simulink model "controller"  (R2023b)
settings: Solver=FixedStepAuto  StartTime=0.0  StopTime=10.0  FixedStep=1/100  RelTol=1e-3
values from neighbouring files (symbols this model uses):
  MAX_TORQUE = 80    [init_fn.m]
  MAX_TORQUE_REVERSE = 40    [init_fn.m]
undefined symbols (not defined in the file or in its folder): MAX_SPEED_BACKWARD, MAX_SPEED_FORWARD
settings Model: Creator=DAUIN-Win10  LastModifiedBy=anton
settings OptimizationCC: ReuseModelBlockBuffer=off
settings DebuggingCC: UnconnectedInputMsg=warning  UnconnectedOutputMsg=warning  UnconnectedLineMsg=warning  UnderSpecifiedDimensionMsg=error
settings ModelReferenceCC: EnableRefExpFcnMdlSchedulingChecks=on
settings RTWCC: DLArmComputeVersion=19.05

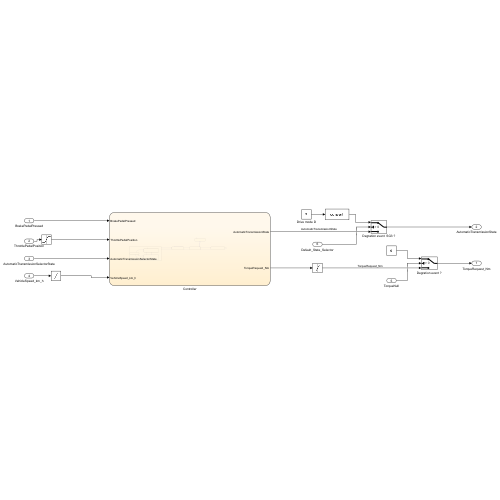
[thumbnail: Simulink's stored preview of the top-level diagram]
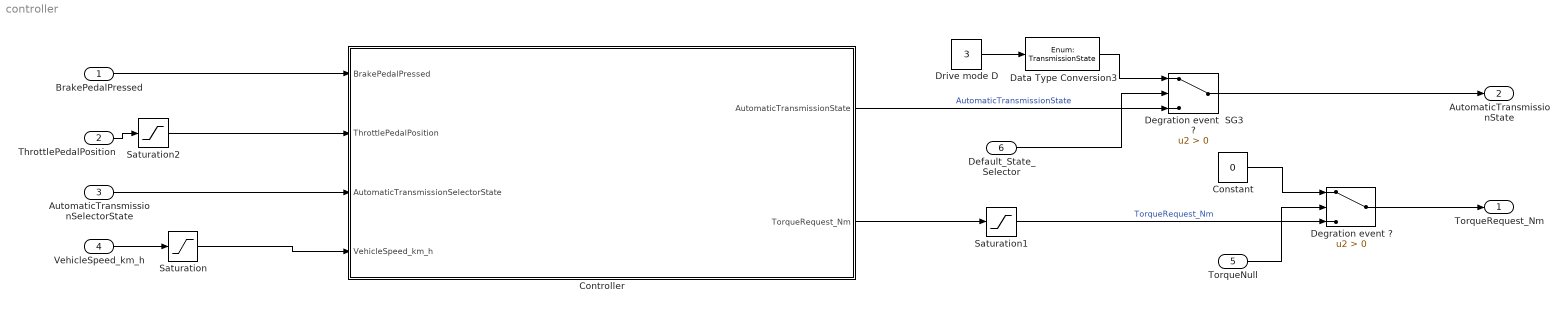
== system controller ==
  BrakePedalPressed : Inport  OutDataTypeStr=boolean
  ThrottlePedalPosition : Inport  Port=2  OutDataTypeStr=single
  AutomaticTransmissionSelectorState : Inport  Port=3  OutDataTypeStr=Enum: TransmissionState
  VehicleSpeed_km_h : Inport  Port=4  OutDataTypeStr=single  Unit=km/h
  TorqueNull : Inport  Port=5
  Default_State_Selector : Inport  Port=6
  Constant : Constant  Value=0  OutDataTypeStr=single
  Controller : Stateflow chart  TreatAsAtomicUnit=on
  Data Type Conversion3 : DataTypeConversion  OutDataTypeStr=Enum: TransmissionState  SaturateOnIntegerOverflow=off  RndMeth=Floor  LockScale=on
  Degration event  SG3 ? : Switch  Criteria=u2 > Threshold  SaturateOnIntegerOverflow=off  InputSameDT=off
  Degration event ? : Switch  Criteria=u2 > Threshold  SaturateOnIntegerOverflow=off  InputSameDT=off
  Drive mode D : Constant  Value=3  OutDataTypeStr=int32
  Saturation : Saturate  UpperLimit=MAX_SPEED_FORWARD  LowerLimit=-MAX_SPEED_BACKWARD
  Saturation1 : Saturate  UpperLimit=MAX_TORQUE  LowerLimit=-MAX_TORQUE_REVERSE
  Saturation2 : Saturate  UpperLimit=1  LowerLimit=0
  TorqueRequest_Nm : Outport  OutDataTypeStr=single  Unit=N*m
  AutomaticTransmissionState : Outport  Port=2  OutDataTypeStr=Enum: TransmissionState
  wires:
  BrakePedalPressed/1 -> Controller/1(BrakePedalPressed)
  VehicleSpeed_km_h/1 -> Saturation/1
  Saturation/1 -> Controller/4(VehicleSpeed_km_h)
  Controller/2(TorqueRequest_Nm) -> Saturation1/1
  ThrottlePedalPosition/1 -> Saturation2/1
  Saturation2/1 -> Controller/2(ThrottlePedalPosition)
  AutomaticTransmissionSelectorState/1 -> Controller/3(AutomaticTransmissionSelectorState)
  TorqueNull/1 -> Degration event ?/2
  Saturation1/1 -> Degration event ?/3  "TorqueRequest_Nm"
  Degration event ?/1 -> TorqueRequest_Nm/1
  Constant/1 -> Degration event ?/1
  Controller/1(AutomaticTransmissionState) -> Degration event  SG3 ?/3  "AutomaticTransmissionState"
  Drive mode D/1 -> Data Type Conversion3/1
  Degration event  SG3 ?/1 -> AutomaticTransmissionState/1
  Default_State_Selector/1 -> Degration event  SG3 ?/2
  Data Type Conversion3/1 -> Degration event  SG3 ?/1

== stateflow chart controller/Controller ==
  state P
    en: AutomaticTransmissionState = TransmissionState.Park;
    exit: TorqueRequest_Nm = 0;
  state B
    entry:
    AutomaticTransmissionState = TransmissionState.Brake;
    state Acceleration
      exit:
      TorqueRequest_Nm = MAX_TORQUE*(ThrottlePedalPosition-1/3)*(3/2)
    state Stopped
      TorqueRequest_Nm= -VehicleSpeed_km_h*50;
    state Braking
      exit:
      TorqueRequest_Nm = -(MAX_TORQUE_REVERSE*(1-(ThrottlePedalPosition*3)))
    (default) -> Acceleration
    Stopped -> Acceleration [order 1] : [ThrottlePedalPosition > 1/3]
    Acceleration -> Acceleration [order 2] : [AutomaticTransmissionSelectorState==TransmissionState.Brake]
    Braking -> Acceleration [order 3] : [ThrottlePedalPosition > 1/3]
    Acceleration -> Braking [order 1] : [ThrottlePedalPosition <= 1/3]
    Braking -> Stopped [order 2] : [ThrottlePedalPosition <=0]
    Stopped -> Braking [order 2] : [VehicleSpeed_km_h > 0]
    Braking -> Braking [order 1] : [AutomaticTransmissionSelectorState==TransmissionState.Brake && VehicleSpeed_km_h >0]
  state R
    entry:
    AutomaticTransmissionState = TransmissionState.Reverse;
    exit:
    TorqueRequest_Nm = -(MAX_TORQUE_REVERSE*ThrottlePedalPosition)
  state D
    entry:
    AutomaticTransmissionState = TransmissionState.Drive;
    exit:
    TorqueRequest_Nm = MAX_TORQUE*ThrottlePedalPosition;
  state N
    entry:
    AutomaticTransmissionState = TransmissionState.Neutral;
    exit:
    TorqueRequest_Nm = 0;
  (default) -> P
  N -> P [order 1] : [(abs(VehicleSpeed_km_h)<5) && BrakePedalPressed==1 && AutomaticTransmissionSelectorState==TransmissionState.Park]
  P -> N : [BrakePedalPressed==1 && (AutomaticTransmissionSelectorState==TransmissionState.Neutral || AutomaticTransmissionSelectorState==TransmissionState.Drive || AutomaticTransmissionSelectorState==TransmissionState.Brake || AutomaticTransmissionSelectorState==TransmissionState.Reverse)]
  D -> D [order 2] : [AutomaticTransmissionSelectorState==TransmissionState.Drive]
  B -> D : [AutomaticTransmissionSelectorState==TransmissionState.Drive]
  R -> R [order 2] : [AutomaticTransmissionSelectorState==TransmissionState.Reverse]
  D -> N [order 3] : [AutomaticTransmissionSelectorState==TransmissionState.Neutral]
  N -> R [order 3] : [VehicleSpeed_km_h<5 && BrakePedalPressed==1 && AutomaticTransmissionSelectorState==TransmissionState.Reverse]
  D -> B [order 1] : [ThrottlePedalPosition>1/3 && AutomaticTransmissionSelectorState==TransmissionState.Brake]
  R -> N [order 1] : [AutomaticTransmissionSelectorState==TransmissionState.Neutral]
  N -> D [order 2] : [VehicleSpeed_km_h>-5 && (AutomaticTransmissionSelectorState==TransmissionState.Drive || AutomaticTransmissionSelectorState==TransmissionState.Brake)]
  data: BrakePedalPressed input boolean size=1; ThrottlePedalPosition input single size=1; AutomaticTransmissionSelectorState input Enum: TransmissionState size=1; VehicleSpeed_km_h input single size=1; AutomaticTransmissionState output Enum: TransmissionState size=1; TorqueRequest_Nm output single size=1; MAX_TORQUE_REVERSE parameter; MAX_TORQUE parameter
